simulink model "SNN_circuit11"  (R2021a)
settings: Solver=FixedStepAuto  StartTime=0.0  StopTime=50  FixedStep=1e-3  RelTol=1e-3
values from neighbouring files (symbols this model uses):
  l = 100e-6    (= 0.0001)    [SNN_run_main11.m]    (also in SNN_run_main22.m; SNN_run_main33.m)
libraries: fl_lib x57, nesl_utility x20, ee_lib x5
(part 2 of 2)

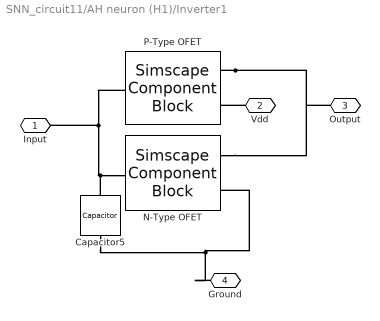
== system SNN_circuit11/AH neuron (H1)/Inverter1 ==
  Capacitor5 : fl_lib/Electrical/Electrical Elements/Capacitor  c=Cgs nF  r=1e-12 Ohm  g=0 1/Ohm  i_specify=off  i_priority=None  i=0 A  i_nominal_specify=off  i_nominal_unit=A  i_nominal_value=1  v_specify=off  v_priority=None  v=0 V  v_nominal_specify=off  v_nominal_unit=V  v_nominal_value=1  vc_specify=off  vc_priority=High  vc=0 V  vc_nominal_specify=off  vc_nominal_unit=V  vc_nominal_value=1
  N-Type OFET : SimscapeComponentBlock  SourceFile=N_Marinov_OFET  ComponentPath=N_Marinov_OFET  ComponentVariants=N_Marinov_OFET  ComponentVariantNames=N_Marinov_OFET  ClassName=N_Marinov_OFET  SchemaVersion=1  Gamma=gama_n  Lambda=landa_n  Vbb=Vbb_n  Vss=Vss_n  aaa=aaa_n  bbb=bbb_n  ccc=ccc_n  Mu0=mu0_n  Vt=Vt_n V  Cox=ci  W=W_n  L=l  i_specify=off  i_priority=None  i=0 A  i_nominal_specify=off  i_nominal_unit=A  i_nominal_value=1  Vgs_specify=off  Vgs_priority=None  Vgs=0 V  Vgs_nominal_specify=off  Vgs_nominal_unit=V  Vgs_nominal_value=1  Vds_specify=off  Vds_priority=None  Vds=0 V  Vds_nominal_specify=off  Vds_nominal_unit=V  Vds_nominal_value=1  Power_specify=off  Power_priority=None  Power=0 W  Power_nominal_specify=off  Power_nominal_unit=W  Power_nominal_value=1
      settings: CopyFcn=simscape.engine.sli.internal.componentblockcallback(gcbh,'COPY')  PreCopyFcn=simscape.engine.sli.internal.componentblockcallback(gcbh,'PRECOPY')  PreDeleteFcn=simscape.engine.sli.internal.componentblockcallback(gcbh,'PREDELETE')  InternalSimscapePortConfiguration="{\"Bottom\":[],\"Left\":[{\"id\":\"g\",\"label\":\"Gate\",\"type\":\"foundation.electrical.electrical\"}],\"Right\":[{\"id\":\"d\",\"label\":\"Drain\",\"type\":\"foundation.electrical.electrical\"},{\"id\":\"s\",\"label\":\"Source\",\"type\":\"foundation.electrical.electrical\"}],\"Top\":[]}"
      mask Type: Marinov OFET
  P-Type OFET : SimscapeComponentBlock  SourceFile=P_Marinov_OFET  ComponentPath=P_Marinov_OFET  ComponentVariants=P_Marinov_OFET  ComponentVariantNames=P_Marinov_OFET  ClassName=P_Marinov_OFET  SchemaVersion=1  Gamma=gama_p  Lambda=landa_p  Vbb=Vbb_p  Vss=Vss_p  aaa=aaa_p  bbb=bbb_p  ccc=ccc_p  Mu0=mu0_p  Vt=Vt_p V  Cox=ci  W=W_p  L=l  i_specify=off  i_priority=None  i=0 A  i_nominal_specify=off  i_nominal_unit=A  i_nominal_value=1  Vsg_specify=off  Vsg_priority=None  Vsg=0 V  Vsg_nominal_specify=off  Vsg_nominal_unit=V  Vsg_nominal_value=1  Vsd_specify=off  Vsd_priority=None  Vsd=0 V  Vsd_nominal_specify=off  Vsd_nominal_unit=V  Vsd_nominal_value=1  Power_specify=off  Power_priority=None  Power=0 W  Power_nominal_specify=off  Power_nominal_unit=W  Power_nominal_value=1
      settings: CopyFcn=simscape.engine.sli.internal.componentblockcallback(gcbh,'COPY')  PreCopyFcn=simscape.engine.sli.internal.componentblockcallback(gcbh,'PRECOPY')  PreDeleteFcn=simscape.engine.sli.internal.componentblockcallback(gcbh,'PREDELETE')  InternalSimscapePortConfiguration="{\"Bottom\":[],\"Left\":[{\"id\":\"g\",\"label\":\"Gate\",\"type\":\"foundation.electrical.electrical\"}],\"Right\":[{\"id\":\"s\",\"label\":\"Source\",\"type\":\"foundation.electrical.electrical\"},{\"id\":\"d\",\"label\":\"Drain\",\"type\":\"foundation.electrical.electrical\"}],\"Top\":[]}"
      mask Type: Marinov OFET
  Input : PMIOPort  Side=Left
  Vdd : PMIOPort  Port=2  Side=Left
  Output : PMIOPort  Port=3  Side=Right
  Ground : PMIOPort  Port=4  Side=Left
  connections:
  Vdd/RConn1 -- P-Type OFET/RConn1
  Ground/RConn1 -- Capacitor5/RConn1 -- N-Type OFET/RConn2
  P-Type OFET/LConn1 -- Input/RConn1 -- N-Type OFET/LConn1 -- Capacitor5/LConn1
  P-Type OFET/RConn2 -- N-Type OFET/RConn1 -- Output/RConn1

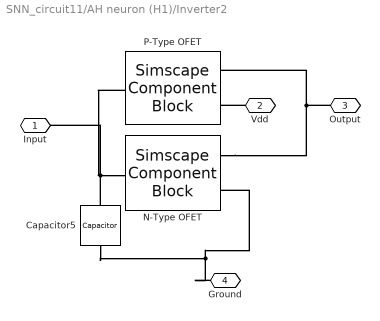
== system SNN_circuit11/AH neuron (H1)/Inverter2 ==
  Capacitor5 : fl_lib/Electrical/Electrical Elements/Capacitor  c=Cgs nF  r=1e-12 Ohm  g=0 1/Ohm  i_specify=off  i_priority=None  i=0 A  i_nominal_specify=off  i_nominal_unit=A  i_nominal_value=1  v_specify=off  v_priority=None  v=0 V  v_nominal_specify=off  v_nominal_unit=V  v_nominal_value=1  vc_specify=off  vc_priority=High  vc=0 V  vc_nominal_specify=off  vc_nominal_unit=V  vc_nominal_value=1
  N-Type OFET : SimscapeComponentBlock  SourceFile=N_Marinov_OFET  ComponentPath=N_Marinov_OFET  ComponentVariants=N_Marinov_OFET  ComponentVariantNames=N_Marinov_OFET  ClassName=N_Marinov_OFET  SchemaVersion=1  Gamma=gama_n  Lambda=landa_n  Vbb=Vbb_n  Vss=Vss_n  aaa=aaa_n  bbb=bbb_n  ccc=ccc_n  Mu0=mu0_n  Vt=Vt_n V  Cox=ci  W=W_n  L=l  i_specify=off  i_priority=None  i=0 A  i_nominal_specify=off  i_nominal_unit=A  i_nominal_value=1  Vgs_specify=off  Vgs_priority=None  Vgs=0 V  Vgs_nominal_specify=off  Vgs_nominal_unit=V  Vgs_nominal_value=1  Vds_specify=off  Vds_priority=None  Vds=0 V  Vds_nominal_specify=off  Vds_nominal_unit=V  Vds_nominal_value=1  Power_specify=off  Power_priority=None  Power=0 W  Power_nominal_specify=off  Power_nominal_unit=W  Power_nominal_value=1
      settings: CopyFcn=simscape.engine.sli.internal.componentblockcallback(gcbh,'COPY')  PreCopyFcn=simscape.engine.sli.internal.componentblockcallback(gcbh,'PRECOPY')  PreDeleteFcn=simscape.engine.sli.internal.componentblockcallback(gcbh,'PREDELETE')  InternalSimscapePortConfiguration="{\"Bottom\":[],\"Left\":[{\"id\":\"g\",\"label\":\"Gate\",\"type\":\"foundation.electrical.electrical\"}],\"Right\":[{\"id\":\"d\",\"label\":\"Drain\",\"type\":\"foundation.electrical.electrical\"},{\"id\":\"s\",\"label\":\"Source\",\"type\":\"foundation.electrical.electrical\"}],\"Top\":[]}"
      mask Type: Marinov OFET
  P-Type OFET : SimscapeComponentBlock  SourceFile=P_Marinov_OFET  ComponentPath=P_Marinov_OFET  ComponentVariants=P_Marinov_OFET  ComponentVariantNames=P_Marinov_OFET  ClassName=P_Marinov_OFET  SchemaVersion=1  Gamma=gama_p  Lambda=landa_p  Vbb=Vbb_p  Vss=Vss_p  aaa=aaa_p  bbb=bbb_p  ccc=ccc_p  Mu0=mu0_p  Vt=Vt_p V  Cox=ci  W=W_p  L=l  i_specify=off  i_priority=None  i=0 A  i_nominal_specify=off  i_nominal_unit=A  i_nominal_value=1  Vsg_specify=off  Vsg_priority=None  Vsg=0 V  Vsg_nominal_specify=off  Vsg_nominal_unit=V  Vsg_nominal_value=1  Vsd_specify=off  Vsd_priority=None  Vsd=0 V  Vsd_nominal_specify=off  Vsd_nominal_unit=V  Vsd_nominal_value=1  Power_specify=off  Power_priority=None  Power=0 W  Power_nominal_specify=off  Power_nominal_unit=W  Power_nominal_value=1
      settings: CopyFcn=simscape.engine.sli.internal.componentblockcallback(gcbh,'COPY')  PreCopyFcn=simscape.engine.sli.internal.componentblockcallback(gcbh,'PRECOPY')  PreDeleteFcn=simscape.engine.sli.internal.componentblockcallback(gcbh,'PREDELETE')  InternalSimscapePortConfiguration="{\"Bottom\":[],\"Left\":[{\"id\":\"g\",\"label\":\"Gate\",\"type\":\"foundation.electrical.electrical\"}],\"Right\":[{\"id\":\"s\",\"label\":\"Source\",\"type\":\"foundation.electrical.electrical\"},{\"id\":\"d\",\"label\":\"Drain\",\"type\":\"foundation.electrical.electrical\"}],\"Top\":[]}"
      mask Type: Marinov OFET
  Input : PMIOPort  Side=Left
  Vdd : PMIOPort  Port=2  Side=Left
  Output : PMIOPort  Port=3  Side=Right
  Ground : PMIOPort  Port=4  Side=Left
  connections:
  N-Type OFET/RConn1 -- Output/RConn1 -- P-Type OFET/RConn2
  Input/RConn1 -- P-Type OFET/LConn1 -- Capacitor5/LConn1 -- N-Type OFET/LConn1
  Ground/RConn1 -- Capacitor5/RConn1 -- N-Type OFET/RConn2
  Vdd/RConn1 -- P-Type OFET/RConn1

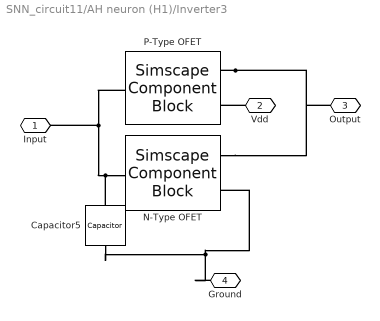
== system SNN_circuit11/AH neuron (H1)/Inverter3 ==
  Capacitor5 : fl_lib/Electrical/Electrical Elements/Capacitor  c=Cgs nF  r=1e-12 Ohm  g=0 1/Ohm  i_specify=off  i_priority=None  i=0 A  i_nominal_specify=off  i_nominal_unit=A  i_nominal_value=1  v_specify=off  v_priority=None  v=0 V  v_nominal_specify=off  v_nominal_unit=V  v_nominal_value=1  vc_specify=off  vc_priority=High  vc=0 V  vc_nominal_specify=off  vc_nominal_unit=V  vc_nominal_value=1
  N-Type OFET : SimscapeComponentBlock  SourceFile=N_Marinov_OFET  ComponentPath=N_Marinov_OFET  ComponentVariants=N_Marinov_OFET  ComponentVariantNames=N_Marinov_OFET  ClassName=N_Marinov_OFET  SchemaVersion=1  Gamma=gama_n  Lambda=landa_n  Vbb=Vbb_n  Vss=Vss_n  aaa=aaa_n  bbb=bbb_n  ccc=ccc_n  Mu0=mu0_n  Vt=Vt_n V  Cox=ci  W=W_n  L=l  i_specify=off  i_priority=None  i=0 A  i_nominal_specify=off  i_nominal_unit=A  i_nominal_value=1  Vgs_specify=off  Vgs_priority=None  Vgs=0 V  Vgs_nominal_specify=off  Vgs_nominal_unit=V  Vgs_nominal_value=1  Vds_specify=off  Vds_priority=None  Vds=0 V  Vds_nominal_specify=off  Vds_nominal_unit=V  Vds_nominal_value=1  Power_specify=off  Power_priority=None  Power=0 W  Power_nominal_specify=off  Power_nominal_unit=W  Power_nominal_value=1
      settings: CopyFcn=simscape.engine.sli.internal.componentblockcallback(gcbh,'COPY')  PreCopyFcn=simscape.engine.sli.internal.componentblockcallback(gcbh,'PRECOPY')  PreDeleteFcn=simscape.engine.sli.internal.componentblockcallback(gcbh,'PREDELETE')  InternalSimscapePortConfiguration="{\"Bottom\":[],\"Left\":[{\"id\":\"g\",\"label\":\"Gate\",\"type\":\"foundation.electrical.electrical\"}],\"Right\":[{\"id\":\"d\",\"label\":\"Drain\",\"type\":\"foundation.electrical.electrical\"},{\"id\":\"s\",\"label\":\"Source\",\"type\":\"foundation.electrical.electrical\"}],\"Top\":[]}"
      mask Type: Marinov OFET
  P-Type OFET : SimscapeComponentBlock  SourceFile=P_Marinov_OFET  ComponentPath=P_Marinov_OFET  ComponentVariants=P_Marinov_OFET  ComponentVariantNames=P_Marinov_OFET  ClassName=P_Marinov_OFET  SchemaVersion=1  Gamma=gama_p  Lambda=landa_p  Vbb=Vbb_p  Vss=Vss_p  aaa=aaa_p  bbb=bbb_p  ccc=ccc_p  Mu0=mu0_p  Vt=Vt_p V  Cox=ci  W=W_p  L=l  i_specify=off  i_priority=None  i=0 A  i_nominal_specify=off  i_nominal_unit=A  i_nominal_value=1  Vsg_specify=off  Vsg_priority=None  Vsg=0 V  Vsg_nominal_specify=off  Vsg_nominal_unit=V  Vsg_nominal_value=1  Vsd_specify=off  Vsd_priority=None  Vsd=0 V  Vsd_nominal_specify=off  Vsd_nominal_unit=V  Vsd_nominal_value=1  Power_specify=off  Power_priority=None  Power=0 W  Power_nominal_specify=off  Power_nominal_unit=W  Power_nominal_value=1
      settings: CopyFcn=simscape.engine.sli.internal.componentblockcallback(gcbh,'COPY')  PreCopyFcn=simscape.engine.sli.internal.componentblockcallback(gcbh,'PRECOPY')  PreDeleteFcn=simscape.engine.sli.internal.componentblockcallback(gcbh,'PREDELETE')  InternalSimscapePortConfiguration="{\"Bottom\":[],\"Left\":[{\"id\":\"g\",\"label\":\"Gate\",\"type\":\"foundation.electrical.electrical\"}],\"Right\":[{\"id\":\"s\",\"label\":\"Source\",\"type\":\"foundation.electrical.electrical\"},{\"id\":\"d\",\"label\":\"Drain\",\"type\":\"foundation.electrical.electrical\"}],\"Top\":[]}"
      mask Type: Marinov OFET
  Input : PMIOPort  Side=Left
  Vdd : PMIOPort  Port=2  Side=Left
  Output : PMIOPort  Port=3  Side=Right
  Ground : PMIOPort  Port=4  Side=Left
  connections:
  Vdd/RConn1 -- P-Type OFET/RConn1
  Ground/RConn1 -- Capacitor5/RConn1 -- N-Type OFET/RConn2
  P-Type OFET/LConn1 -- Input/RConn1 -- Capacitor5/LConn1 -- N-Type OFET/LConn1
  P-Type OFET/RConn2 -- N-Type OFET/RConn1 -- Output/RConn1
